simulink model "tarea0"  (R2025a)
settings: Solver=VariableStepAuto  StartTime=0.0  StopTime=10.0  RelTol=1e-3
InitFcn:
  | I_p=0.0079;
  | M_c=0.7031;
  | L_p=0.3302;
  | M_p=0.23;
  | F_c=0;
  | B_eq=4.3;
  | g=9.81;
  | B_p=0.0024;
settings Model: LastModifiedBy=USER

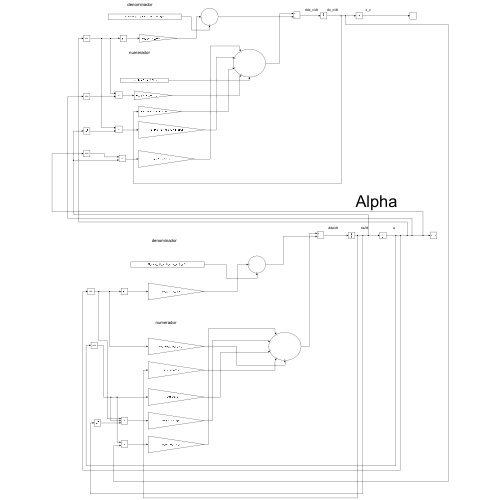
[thumbnail: Simulink's stored preview of the top-level diagram]
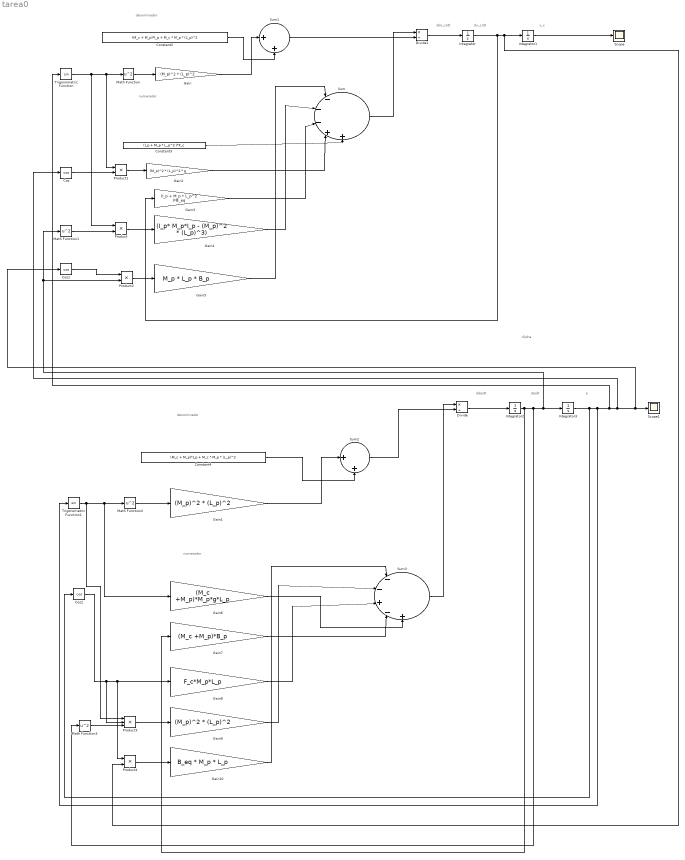
== system tarea0 ==
  note: denominador
  note: Alpha
  note: ddx_c/dt
  note: dx_c/dt
  note: x_c
  note: numerador
  note: denominador
  note: numerador
  note: dda/dt
  note: da/dt
  note: a
  Constant2 : Constant  Value=(M_c + M_p)*I_p + M_c * M_p * (L_p)^2
  Constant3 : Constant  Value=(I_p + M_p * L_p^2 )*F_c
  Constant4 : Constant  Value=(M_c + M_p)*I_p + M_c * M_p * (L_p)^2
  Cos : Trigonometry  Operator=cos
  Cos1 : Trigonometry  Operator=cos
  Cos2 : Trigonometry  Operator=cos
  Divide : Product  Inputs=*/
  Divide1 : Product  Inputs=*/
  Gain : Gain  Gain=(M_p)^2 * (L_p)^2
  Gain1 : Gain  Gain=(M_p)^2 * (L_p)^2
  Gain10 : Gain  Gain=B_eq * M_p * L_p
  Gain2 : Gain  Gain=(M_p)^2 * (L_p)^2 * g
  Gain3 : Gain  Gain=(I_p + M_p * L_p^2 )*B_eq
  Gain4 : Gain  Gain=(I_p* M_p*I_p - (M_p)^2 * (L_p)^3)
  Gain5 : Gain  Gain=M_p * L_p * B_p
  Gain6 : Gain  Gain=(M_c +M_p)*M_p*g*L_p
  Gain7 : Gain  Gain=(M_c +M_p)*B_p
  Gain8 : Gain  Gain=F_c*M_p*L_p
  Gain9 : Gain  Gain=(M_p)^2 * (L_p)^2
  Integrator : Integrator
  Integrator1 : Integrator
  Integrator2 : Integrator
  Integrator3 : Integrator  InitialCondition=1
  Math Function{,1..3} (4 alike) : Math  Operator=square
  Product{,1..2,4} (4 alike) : Product
  Product3 : Product  Inputs=3
  Scope : Scope
      settings: ActiveDisplayYMinimum=-0.25129288699875085  ActiveDisplayYMaximum=0.17464549664003817
  Scope1 : Scope
      settings: ActiveDisplayYMinimum=-84.016901148439914  ActiveDisplayYMaximum=16.040862531966415
  Sum : Sum  Inputs=|---++
  Sum1 : Sum  Inputs=|++
  Sum2 : Sum  Inputs=|++
  Sum3 : Sum  Inputs=|--+-+
  Trigonometric Function : Trigonometry
  Trigonometric Function1 : Trigonometry
  wires:
  Integrator/1 -> Integrator1/1, Product4/2, Gain3/1
  Integrator1/1 -> Scope/1
  Constant2/1 -> Sum1/2
  Trigonometric Function/1 -> Product/1, Product1/1, Math Function/1
  Math Function/1 -> Gain/1
  Integrator2/1 -> Math Function3/1, Product2/2, Math Function1/1, Integrator3/1, Gain7/1
  Integrator3/1 -> Cos2/1, Trigonometric Function/1, Cos/1, Scope1/1, Cos1/1, Trigonometric Function1/1
  Divide/1 -> Integrator2/1
  Cos/1 -> Product1/2
  Product1/1 -> Gain2/1
  Math Function1/1 -> Product/2
  Product/1 -> Gain4/1
  Product2/1 -> Gain5/1
  Divide1/1 -> Integrator/1
  Sum1/1 -> Divide1/2
  Sum/1 -> Divide1/1
  Trigonometric Function1/1 -> Product3/1, Gain6/1, Math Function2/1
  Math Function2/1 -> Gain1/1
  Constant4/1 -> Sum2/2
  Cos2/1 -> Product3/2, Product4/1, Gain8/1
  Math Function3/1 -> Product3/3
  Product3/1 -> Gain9/1
  Product4/1 -> Gain10/1
  Sum3/1 -> Divide/1
  Sum2/1 -> Divide/2
  Cos1/1 -> Product2/1
  Gain1/1 -> Sum2/1
  Gain/1 -> Sum1/1
  Gain6/1 -> Sum3/5
  Gain7/1 -> Sum3/4
  Gain8/1 -> Sum3/3
  Gain9/1 -> Sum3/2
  Gain10/1 -> Sum3/1
  Constant3/1 -> Sum/5
  Gain2/1 -> Sum/4
  Gain3/1 -> Sum/3
  Gain4/1 -> Sum/2
  Gain5/1 -> Sum/1
